simulink library "ddm"  (R2021b)
settings: Solver=VariableStepAuto  StartTime=0.0  StopTime=10.0  RelTol=1e-3
undefined symbols (not defined in the file or in its folder): ENUM_ADASACCSTA_ERROR, ENUM_ADASACCSTA_OFF, ENUM_ADASACCSTA_STANDBY, ENUM_ADASISASTA_OFF, ENUM_ALLOWMOV_ALLOWREADY, ENUM_APS, ENUM_BRKSTA_ERROR, ENUM_BRKSTA_OFF, ENUM_BRKSTA_ON, ENUM_CHGPREACTERRSTA_OBCPRE, ENUM_DCDCFAULTSTA_ANYFAULTLV1, ENUM_DCDCFAULTSTA_ANYFAULTLV2, ENUM_DRIVETRAIN_AWD, ENUM_DRIVETRAIN_FWD, ENUM_DRIVETRAIN_RWD, ENUM_DRSEATSTA_INVALID, ENUM_EDUDRTSTA_NORMAL, ENUM_EPBSTA_APPLIED, ENUM_EPBSTA_RELEASED, ENUM_HVBATTREADYPRE_READY, ENUM_MCUWARN_LV0, ENUM_MCUWARN_LV1, ENUM_MCUWARN_LV2, ENUM_MCUWARN_LV3, ENUM_MCUWARN_NOERROR, ENUM_OBCFAULTSTA_ANYFAULT, ENUM_PAS_R2F2, ENUM_PDFAULT_BATTPDFAIL, ENUM_PDFAULT_DCDCDISABLE, ENUM_PDFAULT_MCUDISABLE, ENUM_PDFAULT_MCUDISCHRG, ENUM_POWERSTA_OFF, ENUM_POWERSTA_ON, ENUM_POWERSTA_READY, ENUM_POWERSTA_STANDBY, ENUM_PRESSINDI_LOW, ENUM_PUFAULT_BATTUPFAIL, ENUM_PUFAULT_DCDCENABLEFAIL, ENUM_PUFAULT_PRECHRGCHKFAIL, ENUM_PUFAULT_SAFETYCHKFAIL, ENUM_PUSTATE_COMPLETED, ENUM_PWRSTASW_OFF, ENUM_PWRSTASW_OFFA, ENUM_PWRSTASW_OFFCHVCHRG, ENUM_PWRSTASW_OFFCLVCHRG, ENUM_PWRSTASW_ON, ENUM_PWRSTASW_ONHVCHRG, ENUM_PWRSTASW_READY, ENUM_PWRSTASW_STANDBY, ENUM_RANGESTA_12IN, ENUM_RANGESTA_12OUT, ENUM_SHIFTCOMMAND_D, ENUM_SHIFTCOMMAND_N, ENUM_SHIFTCOMMAND_P, ENUM_SHIFTCOMMAND_R, ENUM_ZONEMALFUNLV_1ST, ENUM_ZONEMALFUNLV_2ND, ENUM_ZONEMALFUNLV_3RD, ENUM_ZONEMALFUNLV_4TH, ENUM_ZONESPDCTRLMODE_ACC ... (+832)
libraries: hcu_lib x738, $bdroot x26, simulink x7
(part 5 of 25)

== system ddm/DDM/DDM/PMM/Brake switch signal abnormal ==
  task_time_s : Inport
  VPMM_PwrStaSW_enum : Inport  Port=2
  VPMM_PowerSta_enum : Inport  Port=3
  VINP_BrakeSWGPIO_flg : Inport  Port=4
  VINP_BrakeLampSW_flg : Inport  Port=5
  VDDM_ESC5NoComCFS_flg : Inport  Port=6
  VDDM_ESC5RCErrCFS_flg : Inport  Port=7
  VDDM_ESC5CSErrCFS_flg : Inport  Port=8
  VINP_DrStdAErrSta_enum : Inport  Port=9
  VINP_BrkSWSta_flg : Inport  Port=10
  VDDM_ESC7NoComCFS_flg : Inport  Port=11
  VDDM_ESC7RCErrCFS_flg : Inport  Port=12
  VDDM_ESC7CSErrCFS_flg : Inport  Port=13
  VINP_BrkPedalPosSta_enum : Inport  Port=14
  VINP_BrkPedalPos_pct : Inport  Port=15
  DTC_clear_request : Inport  Port=16
  Brake switch signal abnormal : Subsystem
  Brake switch signal abnormal and no backup signal : Subsystem
  Constant : Constant  Value=FALSE
  Constant1 : Constant  Value=ENUM_BRKSTA_ERROR
  Constant2 : Constant  Value=ENUM_BRKSTA_ON
  Constant3 : Constant  Value=ENUM_BRKSTA_OFF
  Constant4 : Constant  Value=FALSE
  Constant5 : Constant  Value=ENUM_BRKSTA_ERROR
  Constant6 : Constant  Value=ENUM_BRKSTA_ON
  Constant7 : Constant  Value=ENUM_BRKSTA_OFF
  Constant8 : Constant  Value=KDDM_BrkPedalPos_pct
  Equal : RelationalOperator  Operator===  OutDataTypeStr=boolean  RndMeth=Simplest
  Equal1 : RelationalOperator  Operator===  OutDataTypeStr=boolean  RndMeth=Simplest
  Equal2 : RelationalOperator  OutDataTypeStr=boolean  RndMeth=Simplest
  Logical Operator : Logic  Operator=OR  Inputs=4  AllPortsSameDT=off  OutDataTypeStr=boolean
  Logical Operator1 : Logic  Operator=OR  Inputs=4  AllPortsSameDT=off  OutDataTypeStr=boolean
  Subsystem : Subsystem
  Switch{,1..3} (4 alike) : Switch  Criteria=u2 > Threshold
  VDDM_BrkSWErrDTC_raw32 : Outport
  VDDM_BrkSWNoBacDTC_raw32 : Outport  Port=2
  VDDM_BrakeSW_enum : Outport  Port=3
  VDDM_CANBrkSW2Sta_enum : Outport  Port=4
  VDDM_BrkPedalPosSta_enum : Outport  Port=5
  VDDM_EDriveSysErrBrake_flg : Outport  Port=6
  VDDM_VCUBrkSWSta_flg : Outport  Port=7
  wires:
  [VPMM_PwrStaSW_enum] -> Brake switch signal abnormal and no backup signal/2(VPMM_PowerSta_enum)
  [VPMM_PowerSta_enum] -> Brake switch signal abnormal and no backup signal/3(VPMM_PwrStaSW_enum)
  [task_time_s] -> Brake switch signal abnormal and no backup signal/1(task_time_s)
  [VPMM_PowerSta_enum] -> Brake switch signal abnormal/3(VPMM_PwrStaSW_enum)
  [VPMM_PwrStaSW_enum] -> Brake switch signal abnormal/2(VPMM_PowerSta_enum)
  [task_time_s] -> Brake switch signal abnormal/1(task_time_s)
  VPMM_PowerSta_enum/1 -> [VPMM_PowerSta_enum]
  VPMM_PwrStaSW_enum/1 -> [VPMM_PwrStaSW_enum]
  task_time_s/1 -> [task_time_s]
  VINP_DrStdAErrSta_enum/1 -> Equal/1
  Constant/1 -> Equal/2
  VDDM_ESC5CSErrCFS_flg/1 -> Logical Operator/3
  VDDM_ESC5RCErrCFS_flg/1 -> Logical Operator/2
  VDDM_ESC5NoComCFS_flg/1 -> Logical Operator/1
  Equal/1 -> Logical Operator/4
  Switch1/1 -> Switch/3
  Logical Operator/1 -> Switch/2
  Constant1/1 -> Switch/1
  VINP_BrkSWSta_flg/1 -> Switch1/2
  Constant2/1 -> Switch1/1
  Constant3/1 -> Switch1/3
  Constant7/1 -> Switch3/3
  Constant6/1 -> Switch3/1
  Constant5/1 -> Switch2/1
  Logical Operator1/1 -> Switch2/2
  Switch3/1 -> Switch2/3
  Equal1/1 -> Logical Operator1/4
  VDDM_ESC7NoComCFS_flg/1 -> Logical Operator1/1
  VDDM_ESC7RCErrCFS_flg/1 -> Logical Operator1/2
  VDDM_ESC7CSErrCFS_flg/1 -> Logical Operator1/3
  Constant4/1 -> Equal1/2
  VINP_BrkPedalPosSta_enum/1 -> Equal1/1
  VINP_BrkPedalPos_pct/1 -> Equal2/1
  Constant8/1 -> Equal2/2
  Equal2/1 -> Switch3/2
  Brake switch signal abnormal/1(VDDM_BrkSWErrDTC_raw32) -> VDDM_BrkSWErrDTC_raw32/1
  Brake switch signal abnormal and no backup signal/1(VDDM_BrkSWNoBacDTC_raw32) -> VDDM_BrkSWNoBacDTC_raw32/1
  Switch/1 -> [VDDM_CANBrkSW2Sta_enum]
  Switch2/1 -> [VDDM_BrkPedalPosSta_enum]
  [VDDM_BrkPedalPosSta_enum] -> VDDM_BrkPedalPosSta_enum/1
  [VDDM_CANBrkSW2Sta_enum] -> VDDM_CANBrkSW2Sta_enum/1
  [VDDM_BrakeSW_enum] -> VDDM_BrakeSW_enum/1
  Brake switch signal abnormal/2(VDDM_EDriveSysErrBrake_flg) -> VDDM_EDriveSysErrBrake_flg/1
  Brake switch signal abnormal and no backup signal/2(VDDM_VCUBrkSWSta_flg) -> VDDM_VCUBrkSWSta_flg/1
  DTC_clear_request/1 -> [DTC_clear_request]
  [DTC_clear_request] -> Brake switch signal abnormal/6(DTC_clear_request)
  [DTC_clear_request] -> Brake switch signal abnormal and no backup signal/6(DTC_clear_request)
  [VDDM_CANBrkSW2Sta_enum] -> Subsystem/1(VDDM_CANBSW2S_enum)
  [VDDM_BrkPedalPosSta_enum] -> Subsystem/4(BrkPedalPos_enum)
  VINP_BrakeSWGPIO_flg/1 -> Subsystem/2(BrakeSW)
  VINP_BrakeLampSW_flg/1 -> Subsystem/3(Brake_Stop_Lamp)
  Subsystem/1(BrkSWErr) -> [BrkSWErr]
  Subsystem/4(VDDM_BrakeSW_enum) -> [VDDM_BrakeSW_enum]  "VDDM_BrakeSW_enum"
  Subsystem/2(BrkSWNoBac) -> [BrkSWNoBac]
  Subsystem/3(BrkSWPass) -> [BrkSWPass]
  [BrkSWErr] -> Brake switch signal abnormal/4(BrkSWErr)
  [BrkSWPass] -> Brake switch signal abnormal/5(BrkSWPass)
  [BrkSWNoBac] -> Brake switch signal abnormal and no backup signal/4(BrkSWNoBac)
  [BrkSWPass] -> Brake switch signal abnormal and no backup signal/5(BrkSWPass)

== system ddm/DDM/DDM/PMM/Comm err ==
  note: CAN1 ABM1
  note: CAN3 CCU2
  note: CAN3 CCU1
  note: CAN3 BMS1
  note: CAN3 BMS6
  note: CAN1 EPAS2
  task_time_s : Inport
  VPMM_PowerSta_enum : Inport  Port=2
  VPMM_PwrStaSW_enum : Inport  Port=3
  VDDM_C3BMS6RCChk_flg : Inport  Port=4
  VDDM_C3BMS6CSChk_flg : Inport  Port=5
  VDDM_C3BMS6LCChk_flg : Inport  Port=6
  VDDM_C3BMS1RCChk_flg : Inport  Port=7
  VDDM_C3BMS1CSChk_flg : Inport  Port=8
  VDDM_C3BMS1LCChk_flg : Inport  Port=9
  VDDM_C3CCU1RCChk_flg : Inport  Port=10
  VDDM_C3CCU1CSChk_flg : Inport  Port=11
  VDDM_C3CCU1LCChk_flg : Inport  Port=12
  VDDM_C3CCU2RCChk_flg : Inport  Port=13
  VDDM_C3CCU2CSChk_flg : Inport  Port=14
  VDDM_C3CCU2LCChk_flg : Inport  Port=15
  VDDM_C1ABM1RCChk_flg : Inport  Port=16
  VDDM_C1ABM1CSChk_flg : Inport  Port=17
  VDDM_C1ABM1LCChk_flg : Inport  Port=18
  No_CAN3_BUS_OFF : Inport  Port=19
  No_CAN1_BUS_OFF : Inport  Port=20
  DTC_clear_request : Inport  Port=21
  VDDM_C1EPAS2LCChk_flg : Inport  Port=22
  FDC lost communication with EPAS2 : Subsystem
  OR : Logic  Operator=OR  Inputs=3  AllPortsSameDT=off  OutDataTypeStr=boolean
  The CAN signal between VCU and ABM1 is discontinuous : Subsystem
  The CAN signal between VCU and ABM1 is incomplete : Subsystem
  The CAN signal between VCU and BMS1 is discontinuous : Subsystem
  The CAN signal between VCU and BMS1 is incomplete : Subsystem
  The CAN signal between VCU and BMS6 is discontinuous : Subsystem
  The CAN signal between VCU and BMS6 is incomplete : Subsystem
  The CAN signal between VCU and CCU1 is discontinuous : Subsystem
  The CAN signal between VCU and CCU1 is incomplete : Subsystem
  The CAN signal between VCU and CCU2 is discontinuous : Subsystem
  The CAN signal between VCU and CCU2 is incomplete : Subsystem
  VCU lost communication with ABM1 : Subsystem
  VCU lost communication with BMS1 : Subsystem
  VCU lost communication with BMS6 : Subsystem
  VCU lost communication with CCU1 : Subsystem
  VCU lost communication with CCU2 : Subsystem
  VDDM_C3BMS6RCDTC_raw32 : Outport
  VDDM_C3BMS6CSDTC_raw32 : Outport  Port=2
  VDDM_C3BMS6LCDTC_raw32 : Outport  Port=3
  VDDM_C3BMS1RCDTC_raw32 : Outport  Port=4
  VDDM_C3BMS1CSDTC_raw32 : Outport  Port=5
  VDDM_C3BMS1LCDTC_raw32 : Outport  Port=6
  VDDM_C3CCU1RCDTC_raw32 : Outport  Port=7
  VDDM_C3CCU1CSDTC_raw32 : Outport  Port=8
  VDDM_C3CCU1LCDTC_raw32 : Outport  Port=9
  VDDM_C3CCU2RCDTC_raw32 : Outport  Port=10
  VDDM_C3CCU2CSDTC_raw32 : Outport  Port=11
  VDDM_C3CCU2LCDTC_raw32 : Outport  Port=12
  VDDM_C1ABM1RCDTC_raw32 : Outport  Port=13
  VDDM_C1ABM1CSDTC_raw32 : Outport  Port=14
  VDDM_C1ABM1LCDTC_raw32 : Outport  Port=15
  VDDM_EDriveSysErrABMCAN_flg : Outport  Port=16
  VDDM_C3BMS6CSCFS_flg : Outport  Port=17
  VDDM_C3BMS6RCCFS_flg : Outport  Port=18
  VDDM_C3BMS6LCCFS_flg : Outport  Port=19
  VDDM_C3CCU2CSCFS_flg : Outport  Port=20
  VDDM_C3CCU2LCCFS_flg : Outport  Port=21
  VDDM_C3CCU2RCCFS_flg : Outport  Port=22
  VDDM_C1EPAS2LCDTC_raw32 : Outport  Port=23
  wires:
  [VDDM_C3CCU2LCCFS_flg] -> The CAN signal between VCU and CCU2 is incomplete/5(VDDM_C3CCU2LCCFS_flg)
  [VPMM_PwrStaSW_enum] -> The CAN signal between VCU and BMS6 is incomplete/3(VPMM_PwrStaSW_enum)
  [VPMM_PwrStaSW_enum] -> VCU lost communication with CCU2/3(VPMM_PwrStaSW_enum)
  [task_time_s] -> VCU lost communication with BMS6/1(task_time_s)
  [task_time_s] -> The CAN signal between VCU and CCU2 is discontinuous/1(task_time_s)
  [task_time_s] -> The CAN signal between VCU and BMS6 is discontinuous/1(task_time_s)
  [VPMM_PwrStaSW_enum] -> VCU lost communication with ABM1/3(VPMM_PwrStaSW_enum)
  VCU lost communication with CCU2/2(VDDM_C3CCU2LCCFS_flg) -> [VDDM_C3CCU2LCCFS_flg]
  [task_time_s] -> VCU lost communication with ABM1/1(task_time_s)
  [task_time_s] -> The CAN signal between VCU and BMS1 is incomplete/1(task_time_s)
  [VPMM_PwrStaSW_enum] -> VCU lost communication with BMS6/3(VPMM_PwrStaSW_enum)
  [VPMM_PowerSta_enum] -> VCU lost communication with ABM1/2(VPMM_PowerSta_enum)
  [VPMM_PwrStaSW_enum] -> The CAN signal between VCU and ABM1 is discontinuous/3(VPMM_PwrStaSW_enum)
  [VPMM_PowerSta_enum] -> The CAN signal between VCU and BMS6 is discontinuous/2(VPMM_PowerSta_enum)
  [task_time_s] -> VCU lost communication with CCU2/1(task_time_s)
  VCU lost communication with ABM1/2(VDDM_C1ABM1LCCFS_flg) -> [VDDM_C1ABM1LCCFS_flg]
  [VPMM_PwrStaSW_enum] -> The CAN signal between VCU and ABM1 is incomplete/3(VPMM_PwrStaSW_enum)
  VDDM_C1ABM1LCChk_flg/1 -> VCU lost communication with ABM1/4(VDDM_C1ABM1LCChk_flg)
  [task_time_s] -> The CAN signal between VCU and BMS6 is incomplete/1(task_time_s)
  [VDDM_C1ABM1LCCFS_flg] -> The CAN signal between VCU and ABM1 is discontinuous/5(VDDM_C1ABM1LCCFS_flg)
  [task_time_s] -> The CAN signal between VCU and CCU1 is incomplete/1(task_time_s)
  VCU lost communication with BMS1/2(VDDM_C3BMS1LCCFS_flg) -> [VDDM_C3BMS1LCCFS_flg]
  [VPMM_PowerSta_enum] -> The CAN signal between VCU and CCU2 is discontinuous/2(VPMM_PowerSta_enum)
  [VPMM_PowerSta_enum] -> VCU lost communication with BMS1/2(VPMM_PowerSta_enum)
  [task_time_s] -> The CAN signal between VCU and BMS1 is discontinuous/1(task_time_s)
  [VPMM_PwrStaSW_enum] -> The CAN signal between VCU and BMS1 is discontinuous/3(VPMM_PwrStaSW_enum)
  [VDDM_C3CCU1LCCFS_flg] -> The CAN signal between VCU and CCU1 is discontinuous/5(VDDM_C3CCU1LCCFS_flg)
  [VPMM_PowerSta_enum] -> The CAN signal between VCU and BMS6 is incomplete/2(VPMM_PowerSta_enum)
  [VDDM_C3CCU2LCCFS_flg] -> The CAN signal between VCU and CCU2 is discontinuous/5(VDDM_C3CCU2LCCFS_flg)
  [VPMM_PwrStaSW_enum] -> VCU lost communication with BMS1/3(VPMM_PwrStaSW_enum)
  [No_CAN3_BUS_OFF] -> The CAN signal between VCU and BMS6 is incomplete/6(No_CAN3_BUS_OFF)
  [VPMM_PowerSta_enum] -> The CAN signal between VCU and BMS1 is discontinuous/2(VPMM_PowerSta_enum)
  [task_time_s] -> The CAN signal between VCU and ABM1 is incomplete/1(task_time_s)
  VDDM_C3BMS1LCChk_flg/1 -> VCU lost communication with BMS1/4(VDDM_C3BMS1LCChk_flg)
  [VPMM_PowerSta_enum] -> The CAN signal between VCU and BMS1 is incomplete/2(VPMM_PowerSta_enum)
  [VDDM_C3BMS1LCCFS_flg] -> The CAN signal between VCU and BMS1 is incomplete/5(VDDM_C3BMS1LCCFS_flg)
  [task_time_s] -> VCU lost communication with CCU1/1(task_time_s)
  [VPMM_PowerSta_enum] -> The CAN signal between VCU and CCU2 is incomplete/2(VPMM_PowerSta_enum)
  [VPMM_PwrStaSW_enum] -> The CAN signal between VCU and BMS1 is incomplete/3(VPMM_PwrStaSW_enum)
  [VPMM_PowerSta_enum] -> VCU lost communication with BMS6/2(VPMM_PowerSta_enum)
  [task_time_s] -> VCU lost communication with BMS1/1(task_time_s)
  [No_CAN3_BUS_OFF] -> The CAN signal between VCU and BMS1 is discontinuous/6(No_CAN3_BUS_OFF)
  VCU lost communication with CCU1/2(VDDM_C3CCU1LCCFS_flg) -> [VDDM_C3CCU1LCCFS_flg]
  [No_CAN3_BUS_OFF] -> The CAN signal between VCU and BMS6 is discontinuous/6(No_CAN3_BUS_OFF)
  [VPMM_PowerSta_enum] -> The CAN signal between VCU and CCU1 is incomplete/2(VPMM_PowerSta_enum)
  [task_time_s] -> The CAN signal between VCU and CCU1 is discontinuous/1(task_time_s)
  [VPMM_PwrStaSW_enum] -> The CAN signal between VCU and BMS6 is discontinuous/3(VPMM_PwrStaSW_enum)
  [VPMM_PwrStaSW_enum] -> The CAN signal between VCU and CCU1 is discontinuous/3(VPMM_PwrStaSW_enum)
  [VPMM_PwrStaSW_enum] -> The CAN signal between VCU and CCU1 is incomplete/3(VPMM_PwrStaSW_enum)
  [VPMM_PowerSta_enum] -> VCU lost communication with CCU1/2(VPMM_PowerSta_enum)
  [VPMM_PwrStaSW_enum] -> VCU lost communication with CCU1/3(VPMM_PwrStaSW_enum)
  [VDDM_C3CCU1LCCFS_flg] -> The CAN signal between VCU and CCU1 is incomplete/5(VDDM_C3CCU1LCCFS_flg)
  [VPMM_PowerSta_enum] -> The CAN signal between VCU and CCU1 is discontinuous/2(VPMM_PowerSta_enum)
  VCU lost communication with BMS6/2(VDDM_C3BMS6LCCFS_flg) -> [VDDM_C3BMS6LCCFS_flg]
  [VPMM_PwrStaSW_enum] -> The CAN signal between VCU and CCU2 is discontinuous/3(VPMM_PwrStaSW_enum)
  [task_time_s] -> The CAN signal between VCU and CCU2 is incomplete/1(task_time_s)
  [VPMM_PowerSta_enum] -> VCU lost communication with CCU2/2(VPMM_PowerSta_enum)
  [VPMM_PowerSta_enum] -> The CAN signal between VCU and ABM1 is incomplete/2(VPMM_PowerSta_enum)
  [VPMM_PwrStaSW_enum] -> The CAN signal between VCU and CCU2 is incomplete/3(VPMM_PwrStaSW_enum)
  [VDDM_C1ABM1LCCFS_flg] -> The CAN signal between VCU and ABM1 is incomplete/5(VDDM_C1ABM1LCCFS_flg)
  [task_time_s] -> The CAN signal between VCU and ABM1 is discontinuous/1(task_time_s)
  [VPMM_PowerSta_enum] -> The CAN signal between VCU and ABM1 is discontinuous/2(VPMM_PowerSta_enum)
  VDDM_C3CCU2CSChk_flg/1 -> The CAN signal between VCU and CCU2 is incomplete/4(VDDM_C3CCU2CSChk_flg)
  VDDM_C3BMS1RCChk_flg/1 -> The CAN signal between VCU and BMS1 is discontinuous/4(VDDM_C3BMS1RCChk_flg)
  VDDM_C3CCU1LCChk_flg/1 -> VCU lost communication with CCU1/4(VDDM_C3CCU1LCChk_flg)
  VDDM_C3CCU1RCChk_flg/1 -> The CAN signal between VCU and CCU1 is discontinuous/4(VDDM_C3CCU1RCChk_flg)
  VDDM_C1ABM1RCChk_flg/1 -> The CAN signal between VCU and ABM1 is discontinuous/4(VDDM_C1ABM1RCChk_flg)
  VDDM_C1ABM1CSChk_flg/1 -> The CAN signal between VCU and ABM1 is incomplete/4(VDDM_C1ABM1CSChk_flg)
  VDDM_C3BMS1CSChk_flg/1 -> The CAN signal between VCU and BMS1 is incomplete/4(VDDM_C3BMS1CSChk_flg)
  VDDM_C3CCU1CSChk_flg/1 -> The CAN signal between VCU and CCU1 is incomplete/4(VDDM_C3CCU1CSChk_flg)
  VDDM_C3CCU2LCChk_flg/1 -> VCU lost communication with CCU2/4(VDDM_C3CCU2LCChk_flg)
  VDDM_C3CCU2RCChk_flg/1 -> The CAN signal between VCU and CCU2 is discontinuous/4(VDDM_C3CCU2RCChk_flg)
  VPMM_PowerSta_enum/1 -> [VPMM_PowerSta_enum]
  VPMM_PwrStaSW_enum/1 -> [VPMM_PwrStaSW_enum]
  task_time_s/1 -> [task_time_s]
  VDDM_C3BMS6RCChk_flg/1 -> The CAN signal between VCU and BMS6 is discontinuous/4(VDDM_C3BMS6RCChk_flg)
  VDDM_C3BMS6CSChk_flg/1 -> The CAN signal between VCU and BMS6 is incomplete/4(VDDM_C3BMS6CSChk_flg)
  VDDM_C3BMS6LCChk_flg/1 -> VCU lost communication with BMS6/4(VDDM_C3BMS6LCChk_flg)
  [DTC_clear_request] -> The CAN signal between VCU and BMS6 is discontinuous/7(DTC_clear_request)
  [DTC_clear_request] -> The CAN signal between VCU and BMS6 is incomplete/7(DTC_clear_request)
  [VDDM_C3BMS6LCCFS_flg] -> The CAN signal between VCU and BMS6 is discontinuous/5(VDDM_C3BMS6LCCFS_flg)
  [VDDM_C3BMS6LCCFS_flg] -> The CAN signal between VCU and BMS6 is incomplete/5(VDDM_C3BMS6LCCFS_flg)
  [No_CAN3_BUS_OFF] -> VCU lost communication with BMS6/5(No_CAN3_BUS_OFF)
  [DTC_clear_request] -> VCU lost communication with BMS6/6(DTC_clear_request)
  [DTC_clear_request] -> The CAN signal between VCU and BMS1 is discontinuous/7(DTC_clear_request)
  [VDDM_C3BMS1LCCFS_flg] -> The CAN signal between VCU and BMS1 is discontinuous/5(VDDM_C3BMS1LCCFS_flg)
  [No_CAN3_BUS_OFF] -> The CAN signal between VCU and BMS1 is incomplete/6(No_CAN3_BUS_OFF)
  [DTC_clear_request] -> The CAN signal between VCU and BMS1 is incomplete/7(DTC_clear_request)
  [No_CAN3_BUS_OFF] -> VCU lost communication with BMS1/5(No_CAN3_BUS_OFF)
  [DTC_clear_request] -> VCU lost communication with BMS1/6(DTC_clear_request)
  [No_CAN3_BUS_OFF] -> The CAN signal between VCU and CCU1 is discontinuous/6(No_CAN3_BUS_OFF)
  [DTC_clear_request] -> The CAN signal between VCU and CCU1 is discontinuous/7(DTC_clear_request)
  [No_CAN3_BUS_OFF] -> The CAN signal between VCU and CCU1 is incomplete/6(No_CAN3_BUS_OFF)
  [DTC_clear_request] -> The CAN signal between VCU and CCU1 is incomplete/7(DTC_clear_request)
  [No_CAN3_BUS_OFF] -> VCU lost communication with CCU1/5(No_CAN3_BUS_OFF)
  [DTC_clear_request] -> VCU lost communication with CCU1/6(DTC_clear_request)
  [No_CAN3_BUS_OFF] -> The CAN signal between VCU and CCU2 is discontinuous/6(No_CAN3_BUS_OFF)
  [DTC_clear_request] -> The CAN signal between VCU and CCU2 is discontinuous/7(DTC_clear_request)
  [No_CAN3_BUS_OFF] -> The CAN signal between VCU and CCU2 is incomplete/6(No_CAN3_BUS_OFF)
  [DTC_clear_request] -> The CAN signal between VCU and CCU2 is incomplete/7(DTC_clear_request)
  [No_CAN3_BUS_OFF] -> VCU lost communication with CCU2/5(No_CAN3_BUS_OFF)
  [DTC_clear_request] -> VCU lost communication with CCU2/6(DTC_clear_request)
  [No_CAN1_BUS_OFF] -> The CAN signal between VCU and ABM1 is discontinuous/6(No_CAN1_BUS_OFF)
  [DTC_clear_request] -> The CAN signal between VCU and ABM1 is discontinuous/7(DTC_clear_request)
  [No_CAN1_BUS_OFF] -> The CAN signal between VCU and ABM1 is incomplete/6(No_CAN1_BUS_OFF)
  [DTC_clear_request] -> The CAN signal between VCU and ABM1 is incomplete/7(DTC_clear_request)
  The CAN signal between VCU and ABM1 is discontinuous/2(RC_EDriveSysErr_VCUErr_flg) -> [VDDM_EDriveSysErrABMRC_flg]
  The CAN signal between VCU and ABM1 is incomplete/2(CS_EDriveSysErr_VCUErr_flg) -> [VDDM_EDriveSysErrABMCS_flg]
  [No_CAN1_BUS_OFF] -> VCU lost communication with ABM1/5(No_CAN1_BUS_OFF)
  [DTC_clear_request] -> VCU lost communication with ABM1/6(DTC_clear_request)
  VCU lost communication with ABM1/3(LC_EDriveSysErr_VCUErr_flg) -> [VDDM_EDriveSysErrABMLC_flg]
  [VDDM_EDriveSysErrABMCS_flg] -> OR/2
  [VDDM_EDriveSysErrABMRC_flg] -> OR/1
  [VDDM_EDriveSysErrABMLC_flg] -> OR/3
  OR/1 -> VDDM_EDriveSysErrABMCAN_flg/1
  No_CAN3_BUS_OFF/1 -> [No_CAN3_BUS_OFF]
  No_CAN1_BUS_OFF/1 -> [No_CAN1_BUS_OFF]
  DTC_clear_request/1 -> [DTC_clear_request]
  The CAN signal between VCU and BMS6 is discontinuous/1(VDDM_C3BMS6RCDTC_raw32) -> VDDM_C3BMS6RCDTC_raw32/1
  The CAN signal between VCU and BMS6 is incomplete/1(VDDM_C3BMS6CSDTC_raw32) -> VDDM_C3BMS6CSDTC_raw32/1
  The CAN signal between VCU and BMS1 is discontinuous/1(VDDM_C3BMS1RCDTC_raw32) -> VDDM_C3BMS1RCDTC_raw32/1
  The CAN signal between VCU and BMS1 is incomplete/1(VDDM_C3BMS1CSDTC_raw32) -> VDDM_C3BMS1CSDTC_raw32/1
  VCU lost communication with BMS1/1(VDDM_C3BMS1LCDTC_raw32) -> VDDM_C3BMS1LCDTC_raw32/1
  The CAN signal between VCU and CCU1 is incomplete/1(VDDM_C3CCU1CSDTC_raw32) -> VDDM_C3CCU1CSDTC_raw32/1
  VCU lost communication with CCU1/1(VDDM_C3CCU1LCDTC_raw32) -> VDDM_C3CCU1LCDTC_raw32/1
  The CAN signal between VCU and CCU2 is discontinuous/1(VDDM_C3CCU2RCDTC_raw32) -> VDDM_C3CCU2RCDTC_raw32/1
  The CAN signal between VCU and CCU2 is incomplete/1(VDDM_C3CCU2CSDTC_raw32) -> VDDM_C3CCU2CSDTC_raw32/1
  VCU lost communication with CCU2/1(VDDM_C3CCU2LCDTC_raw32) -> VDDM_C3CCU2LCDTC_raw32/1
  The CAN signal between VCU and ABM1 is discontinuous/1(VDDM_C1ABM1RCDTC_raw32) -> VDDM_C1ABM1RCDTC_raw32/1
  The CAN signal between VCU and ABM1 is incomplete/1(VDDM_C1ABM1CSDTC_raw32) -> VDDM_C1ABM1CSDTC_raw32/1
  VCU lost communication with ABM1/1(VDDM_C1ABM1LCDTC_raw32) -> VDDM_C1ABM1LCDTC_raw32/1
  VCU lost communication with BMS6/1(VDDM_C3BMS6LCDTC_raw32) -> VDDM_C3BMS6LCDTC_raw32/1
  The CAN signal between VCU and CCU1 is discontinuous/1(VDDM_C3CCU1RCDTC_raw32) -> VDDM_C3CCU1RCDTC_raw32/1
  The CAN signal between VCU and BMS6 is incomplete/2(VDDM_C3BMS6CSCFS_flg) -> VDDM_C3BMS6CSCFS_flg/1
  [VDDM_C3BMS6LCCFS_flg] -> VDDM_C3BMS6LCCFS_flg/1
  The CAN signal between VCU and BMS6 is discontinuous/2(VDDM_C3BMS6RCCFS_flg) -> VDDM_C3BMS6RCCFS_flg/1
  The CAN signal between VCU and CCU2 is incomplete/2(VDDM_C3CCU2CSCFS_flg) -> VDDM_C3CCU2CSCFS_flg/1
  [VDDM_C3CCU2LCCFS_flg] -> VDDM_C3CCU2LCCFS_flg/1
  The CAN signal between VCU and CCU2 is discontinuous/2(VDDM_C3CCU2RCCFS_flg) -> VDDM_C3CCU2RCCFS_flg/1
  FDC lost communication with EPAS2/1(VDDM_C1EPAS2LCDTC_raw32) -> VDDM_C1EPAS2LCDTC_raw32/1
  [DTC_clear_request] -> FDC lost communication with EPAS2/6(DTC_clear_request)
  [No_CAN1_BUS_OFF] -> FDC lost communication with EPAS2/5(No_CAN1_BUS_OFF)
  VDDM_C1EPAS2LCChk_flg/1 -> FDC lost communication with EPAS2/4(VDDM_C1EPAS2LCChk_flg)
  [VPMM_PwrStaSW_enum] -> FDC lost communication with EPAS2/3(VPMM_PwrStaSW_enum)
  [VPMM_PowerSta_enum] -> FDC lost communication with EPAS2/2(VPMM_PowerSta_enum)
  FDC lost communication with EPAS2/2(VDDM_C1EPAS2LCCFS_flg) -> [VDDM_C1EPAS2LCCFS_flg]
  [task_time_s] -> FDC lost communication with EPAS2/1(task_time_s)

== system ddm/DDM/DDM/PMM/Fault level ==
  task_time_s : Inport
  VPMM_PwrStaSW_enum : Inport  Port=2
  VPMM_PowerSta_enum : Inport  Port=3
  VINP_BMSWarn1_flg : Inport  Port=4
  VINP_BMSWarn2_flg : Inport  Port=5
  VINP_BMSWarn3_flg : Inport  Port=6
  VINP_BMSWarn4_flg : Inport  Port=7
  VINP_BMSWarn5_flg : Inport  Port=8
  VINP_BMSWarn6_flg : Inport  Port=9
  VINP_BMSWarn7_flg : Inport  Port=10
  VINP_BMSWarn8_flg : Inport  Port=11
  VINP_DCDCFaultSta_enum : Inport  Port=12
  VPMM_DrivetrainSelect_enum : Inport  Port=13
  VDDM_C3BMS6LCCFS_flg : Inport  Port=14
  VDDM_C3CCU2LCCFS_flg : Inport  Port=15
  VDDM_MCUF1NoComCFS_flg : Inport  Port=16
  VDDM_MCUR1NoComCFS_flg : Inport  Port=17
  VINP_MCUWarnF_enum : Inport  Port=18
  VINP_MCUWarnR_enum : Inport  Port=19
  VINP_OBCFaultSta_enum : Inport  Port=20
  DTC_clear_request : Inport  Port=21
  No_CAN3_BUS_OFF : Inport  Port=22
  Fault level 1 subsystem error : Subsystem
  Fault level 2 subsystem error : Subsystem
  Fault level 3 subsystem error : Subsystem
  Fault level 4 subsystem error : Subsystem
  VDDM_Lv1ErrDTC_raw32 : Outport
  VDDM_Lv2ErrCFS_flg : Outport  Port=2
  VDDM_Lv3ErrDTC_raw32 : Outport  Port=3
  VDDM_Lv4ErrDTC_raw32 : Outport  Port=4
  wires:
  task_time_s/1 -> [task_time_s]
  VPMM_PwrStaSW_enum/1 -> [VPMM_PwrStaSW_enum]
  VPMM_PowerSta_enum/1 -> [VPMM_PowerSta_enum]
  [task_time_s] -> Fault level 1 subsystem error/1(task_time_s)
  [VPMM_PwrStaSW_enum] -> Fault level 1 subsystem error/2(VPMM_PowerSta_enum)
  [VPMM_PowerSta_enum] -> Fault level 1 subsystem error/3(VPMM_PwrStaSW_enum)
  [VPMM_PowerSta_enum] -> Fault level 2 subsystem error/3(VPMM_PwrStaSW_enum)
  [VPMM_PwrStaSW_enum] -> Fault level 2 subsystem error/2(VPMM_PowerSta_enum)
  [task_time_s] -> Fault level 2 subsystem error/1(task_time_s)
  VINP_DCDCFaultSta_enum/1 -> [VINP_DCDCFaultSta_enum]
  [VINP_DCDCFaultSta_enum] -> Fault level 2 subsystem error/10(VINP_DCDCFaultSta_enum)
  [VINP_DCDCFaultSta_enum] -> Fault level 1 subsystem error/11(VINP_DCDCFaultSta_enum)
  [task_time_s] -> Fault level 3 subsystem error/1(task_time_s)
  [VPMM_PwrStaSW_enum] -> Fault level 3 subsystem error/2(VPMM_PowerSta_enum)
  [VPMM_PowerSta_enum] -> Fault level 3 subsystem error/3(VPMM_PwrStaSW_enum)
  VPMM_DrivetrainSelect_enum/1 -> [VPMM_DrivetrainSelect_enum]
  [VPMM_DrivetrainSelect_enum] -> Fault level 1 subsystem error/15(VPMM_DrivetrainSelect_enum)
  [task_time_s] -> Fault level 4 subsystem error/1(task_time_s)
  [VPMM_PwrStaSW_enum] -> Fault level 4 subsystem error/2(VPMM_PowerSta_enum)
  [VPMM_PowerSta_enum] -> Fault level 4 subsystem error/3(VPMM_PwrStaSW_enum)
  VDDM_C3BMS6LCCFS_flg/1 -> [VDDM_C3BMS6LCCFS_flg]
  [VDDM_C3BMS6LCCFS_flg] -> Fault level 1 subsystem error/4(VDDM_C3BMS6LCCFS_flg)
  [VDDM_C3BMS6LCCFS_flg] -> Fault level 2 subsystem error/4(VDDM_C3BMS6LCCFS_flg)
  VDDM_MCUR1NoComCFS_flg/1 -> [VDDM_MCUR1NoComCFS_flg]
  VDDM_MCUF1NoComCFS_flg/1 -> [VDDM_MCUF1NoComCFS_flg]
  [VDDM_MCUR1NoComCFS_flg] -> Fault level 1 subsystem error/7(VDDM_MCUR1NoComCFS_flg)
  [VDDM_MCUF1NoComCFS_flg] -> Fault level 1 subsystem error/6(VDDM_MCUF1NoComCFS_flg)
  VINP_BMSWarn5_flg/1 -> Fault level 2 subsystem error/9(VINP_BMSWarn5_flg)
  VINP_BMSWarn4_flg/1 -> Fault level 2 subsystem error/8(VINP_BMSWarn4_flg)
  [VDDM_MCUR1NoComCFS_flg] -> Fault level 2 subsystem error/7(VDDM_MCUR1NoComCFS_flg)
  [VDDM_MCUF1NoComCFS_flg] -> Fault level 2 subsystem error/6(VDDM_MCUF1NoComCFS_flg)
  [VDDM_MCUF1NoComCFS_flg] -> Fault level 3 subsystem error/5(VDDM_MCUF1NoComCFS_flg)
  [VDDM_MCUR1NoComCFS_flg] -> Fault level 3 subsystem error/6(VDDM_MCUR1NoComCFS_flg)
  [VDDM_C3BMS6LCCFS_flg] -> Fault level 3 subsystem error/4(VDDM_C3BMS6LCCFS_flg)
  [VDDM_C3BMS6LCCFS_flg] -> Fault level 4 subsystem error/4(VDDM_C3BMS6LCCFS_flg)
  VINP_BMSWarn7_flg/1 -> Fault level 4 subsystem error/5(VINP_BMSWarn7_flg)
  VINP_BMSWarn8_flg/1 -> Fault level 4 subsystem error/6(VINP_BMSWarn8_flg)
  VINP_BMSWarn6_flg/1 -> Fault level 3 subsystem error/7(VINP_BMSWarn6_flg)
  VDDM_C3CCU2LCCFS_flg/1 -> [VDDM_C3CCU2LCCFS_flg]
  [VDDM_C3CCU2LCCFS_flg] -> Fault level 1 subsystem error/5(VDDM_C3CCU2LCCFS_flg)
  [VDDM_C3CCU2LCCFS_flg] -> Fault level 2 subsystem error/5(VDDM_C3CCU2LCCFS_flg)
  VINP_BMSWarn1_flg/1 -> Fault level 1 subsystem error/8(VINP_BMSWarn1_flg)
  VINP_BMSWarn2_flg/1 -> Fault level 1 subsystem error/9(VINP_BMSWarn2_flg)
  VINP_BMSWarn3_flg/1 -> Fault level 1 subsystem error/10(VINP_BMSWarn3_flg)
  VINP_MCUWarnF_enum/1 -> [VINP_MCUWarnF_enum]
  VINP_MCUWarnR_enum/1 -> [VINP_MCUWarnR_enum]
  VINP_OBCFaultSta_enum/1 -> [VINP_OBCFaultSta_enum]
  [VINP_OBCFaultSta_enum] -> Fault level 1 subsystem error/14(VINP_OBCFaultSta_enum)
  [VPMM_DrivetrainSelect_enum] -> Fault level 2 subsystem error/13(VPMM_DrivetrainSelect_enum)
  [VINP_MCUWarnF_enum] -> Fault level 2 subsystem error/11(VINP_MCUWarnF_enum)
  [VINP_MCUWarnR_enum] -> Fault level 2 subsystem error/12(VINP_MCUWarnR_enum)
  [VPMM_DrivetrainSelect_enum] -> Fault level 3 subsystem error/10(VPMM_DrivetrainSelect_enum)
  [VINP_MCUWarnR_enum] -> Fault level 3 subsystem error/9(VINP_MCUWarnR_enum)
  [VINP_MCUWarnF_enum] -> Fault level 3 subsystem error/8(VINP_MCUWarnF_enum)
  Fault level 1 subsystem error/1(VDDM_Lv1ErrDTC_raw32) -> VDDM_Lv1ErrDTC_raw32/1
  Fault level 2 subsystem error/1(VDDM_Lv2ErrDTC_raw32) -> VDDM_Lv2ErrCFS_flg/1
  Fault level 3 subsystem error/1(VDDM_Lv3ErrDTC_raw32) -> VDDM_Lv3ErrDTC_raw32/1
  Fault level 4 subsystem error/1(VDDM_Lv4ErrDTC_raw32) -> VDDM_Lv4ErrDTC_raw32/1
  [VINP_MCUWarnF_enum] -> Fault level 1 subsystem error/12(VINP_MCUWarnF_enum)
  [VINP_MCUWarnR_enum] -> Fault level 1 subsystem error/13(VINP_MCUWarnR_enum)
  No_CAN3_BUS_OFF/1 -> [No_CAN3_BUS_OFF]
  DTC_clear_request/1 -> [DTC_clear_request]
  [No_CAN3_BUS_OFF] -> Fault level 1 subsystem error/17(No_CAN3_BUS_OFF)
  [DTC_clear_request] -> Fault level 1 subsystem error/16(DTC_clear_request)
  [DTC_clear_request] -> Fault level 2 subsystem error/14(DTC_clear_request)
  [No_CAN3_BUS_OFF] -> Fault level 2 subsystem error/15(No_CAN3_BUS_OFF)
  [No_CAN3_BUS_OFF] -> Fault level 3 subsystem error/12(No_CAN3_BUS_OFF)
  [DTC_clear_request] -> Fault level 3 subsystem error/11(DTC_clear_request)
  [DTC_clear_request] -> Fault level 4 subsystem error/7(DTC_clear_request)
  [No_CAN3_BUS_OFF] -> Fault level 4 subsystem error/8(No_CAN3_BUS_OFF)

== system ddm/DDM/DDM/PMM/Key authentication failed ==
  note: Fail Safe Operation During Failure Detection
  note: Test Pass Criteria
  note: Diagnostics and Fault Handling
  note: Release Condition After Failure Decision
  note: Test Detection Criteria
  note: Fail Safe Operation After Failure Decision
  note: Release Condition During Failure Detection
  task_time_s : Inport
  VPMM_PowerSta_enum : Inport  Port=2
  VPMM_PwrStaSW_enum : Inport  Port=3
  VDDM_BrakeSW_enum : Inport  Port=4
  DTC_clear_request : Inport  Port=5
  VDKC_DKCAuthSta_enum : Inport  Port=6
  Constant11 : Constant  Value=KDDM_KeyAuthPassSW_flg
  Constant15 : Constant  Value=KDDM_KeyAuthCFSSW_flg
  Constant16 : Constant  Value=TRUE
  Constant19 : Constant  Value=ENUM_POWERSTA_OFF
  Constant{2,21,25,27} (4 alike) : Constant  Value=FALSE
  Constant20 : Constant  Value=KDDM_KeyAuthDFSSW_flg
  Constant23 : Constant  Value=TRUE
  Constant24 : Constant  Value=TRUE
  Constant26 : Constant  Value=ENUM_PWRSTASW_READY
  Constant3 : Constant  Value=ENUM_BRKSTA_ON
  Constant38 : Constant  Value=KDDM_KeyAuthDetTO_s
  Constant4 : Constant  Value=ENUM_PWRSTASW_READY
  Constant40 : Constant  Value=KDDM_KeyAuthDTC_cnt
  Constant43 : Constant  Value=KDDM_KeyAuthPassTO_s
  Constant44 : Constant  Value=KDDM_KeyAuthDetSW_flg
  Constant5 : Constant  Value=ENUM_BRKSTA_ON
  Constant7 : Constant  Value=KDDM_KeyAuthPassTO_s
  Constant8 : Constant  Value=KDDM_KeyAuthDTC_cnt
  DTC_Couter : hcu_lib/Basic_Blocks/DTC_Couter
  DTC_Info : hcu_lib/Basic_Blocks/DTC_Info
  Data Type Conversion1 : DataTypeConversion  OutDataTypeStr=uint8
  Equal{,2..3,5..6} (5 alike) : RelationalOperator  Operator===  OutDataTypeStr=boolean  RndMeth=Simplest
  Equal4 : RelationalOperator  OutDataTypeStr=boolean  RndMeth=Simplest
  Logical Operator{1..2,12,15,18..19} (6 alike) : Logic  AllPortsSameDT=off  OutDataTypeStr=boolean
  Logical Operator3 : Logic  Operator=OR  AllPortsSameDT=off  OutDataTypeStr=boolean
  Logical Operator6 : Logic  Operator=NOT  AllPortsSameDT=off  OutDataTypeStr=boolean
  Logical Operator8 : Logic  Operator=OR  AllPortsSameDT=off  OutDataTypeStr=boolean
  Relay : Relay  OnSwitchValue=ONE_INT  OffSwitchValue=ZERO_INT
  SR_Latch1 : Subsystem  mask(SR_Latch){}
      mask help: SR latch function.
  SR_Latch3 : hcu_lib/Basic_Blocks/SR_Latch
  SR_Latch4 : hcu_lib/Basic_Blocks/SR_Latch
  Switch{,2,4..6} (5 alike) : Switch  Criteria=u2 ~= 0
  Test Detection Criteria : hcu_lib/Basic_Blocks/Test Detection Criteria
  Timer1 : hcu_lib/Basic_Blocks/Timer
  VDDM_KeyAuthDTC_raw32 : Outport
  VDDM_EDriveSysErrKeyAuth_flg : Outport  Port=2
  wires:
  VPMM_PowerSta_enum/1 -> [VPMM_PowerSta_enum]
  VPMM_PwrStaSW_enum/1 -> [VPMM_PwrStaSW_enum]
  task_time_s/1 -> [task_time_s]
  VDDM_BrakeSW_enum/1 -> [VDDM_BrakeSW_enum]
  VDKC_DKCAuthSta_enum/1 -> [VDKC_DKCAuthSta_enum]
  Timer1/1 -> Equal4/1
  [VPMM_PwrStaSW_enum] -> Equal/1
  [task_time_s] -> Test Detection Criteria/2
  [VDDM_KeyAuthDTC_cnt] -> Relay/1
  Logical Operator3/1 -> Logical Operator15/1
  Constant40/1 -> Test Detection Criteria/3
  Constant43/1 -> Timer1/4
  Constant26/1 -> Equal/2
  Constant15/1 -> Logical Operator18/2
  Constant11/1 -> Logical Operator15/2
  Data Type Conversion1/1 -> [VDDM_KeyAuthDTC_cnt]  "VDDM_KeyAuthDTC_cnt"
  Logical Operator15/1 -> DTC_Couter/2
  Logical Operator6/1 -> Timer1/1
  Logical Operator12/1 -> [VDDM_KeyAuthDFS_flg]
  SR_Latch1/1(latched) -> [VDDM_KeyAuthPass_flg]
  [VDDM_KeyAuthCFS_flg] -> Switch/2
  Constant27/1 -> Switch5/3
  Constant24/1 -> Switch4/1
  Logical Operator19/1 -> DTC_Couter/1
  Equal/1 -> Logical Operator2/1
  Switch2/1 -> Timer1/2, Logical Operator6/1
  Logical Operator18/1 -> [VDDM_KeyAuthCFS_flg]
  [VDDM_KeyAuthCFSRls_flg] -> Logical Operator3/2
  Switch/1 -> [VDDM_EDriveSysErrKeyAuth_flg]
  DTC_Couter/2 -> Data Type Conversion1/1
  [VDDM_KeyAuthPass_flg] -> Logical Operator3/1
  [VPMM_PowerSta_enum] -> Equal5/1
  Constant16/1 -> Switch/1
  Logical Operator2/1 -> Switch5/2
  DTC_Couter/1 -> SR_Latch4/1
  Constant19/1 -> Equal5/2
  Logical Operator8/1 -> Switch4/2
  Switch4/1 -> [VDDM_KeyAuthCFSRls_flg]
  [VDDM_KeyAuthDet_flg] -> Logical Operator19/1
  Relay/1 -> SR_Latch3/1
  Constant21/1 -> Switch/3
  Constant20/1 -> Logical Operator12/1
  Test Detection Criteria/1 -> [VDDM_KeyAuthDet_flg]  "VDDM_KeyAuthDet_flg"
  SR_Latch4/1 -> Logical Operator18/1
  Constant8/1 -> DTC_Couter/3
  Constant25/1 -> Switch4/3
  Equal4/1 -> SR_Latch1/1(set)
  Constant44/1 -> Logical Operator19/2
  Constant7/1 -> Equal4/2
  Constant23/1 -> Switch2/3
  SR_Latch3/1 -> Logical Operator12/2
  Equal5/1 -> Logical Operator8/1
  [VDDM_KeyAuthCFSRls_flg] -> SR_Latch4/2
  [DTC_clear_request] -> Logical Operator8/2
  Equal2/1 -> Logical Operator2/2
  [VDDM_BrakeSW_enum] -> Equal2/1
  Constant3/1 -> Equal2/2
  [VDKC_DKCAuthSta_enum] -> Switch5/1
  [VPMM_PwrStaSW_enum] -> Equal3/1
  Equal3/1 -> Logical Operator1/1
  Logical Operator1/1 -> Switch2/2
  [VDDM_BrakeSW_enum] -> Equal6/1
  Constant5/1 -> Equal6/2
  [VDKC_DKCAuthSta_enum] -> Switch2/1
  Equal6/1 -> Logical Operator1/2
  Constant4/1 -> Equal3/2
  DTC_clear_request/1 -> [DTC_clear_request]
  [VDDM_EDriveSysErrKeyAuth_flg] -> VDDM_EDriveSysErrKeyAuth_flg/1
  [task_time_s] -> Timer1/3
  [VDDM_KeyAuthPass_flg] -> DTC_Info/2
  [VDDM_KeyAuthCFS_flg] -> DTC_Info/3
  DTC_Info/1 -> VDDM_KeyAuthDTC_raw32/1  "VDDM_KeyAuthDTC_raw32"
  [VDDM_KeyAuthCFS_flg] -> SR_Latch3/2
  [VDDM_KeyAuthDet_flg] -> DTC_Info/1
  Constant38/1 -> Test Detection Criteria/4
  [DTC_clear_request] -> DTC_Info/4
  [DTC_clear_request] -> Switch6/2
  Switch6/1 -> Test Detection Criteria/1
  Switch5/1 -> [VDDM_xxx_flg], Switch6/3
  Constant2/1 -> Switch6/1
  [VDDM_xxx_flg] -> SR_Latch1/2(reset)

== system ddm/DDM/DDM/PMM/LV ==
  task_time_s : Inport
  VPMM_PwrStaSW_enum : Inport  Port=2
  VPMM_PowerSta_enum : Inport  Port=3
  VINP_LVBattDet12V_V : Inport  Port=4
  VINP_CANMsgValidBMS2_flg : Inport  Port=5
  DTC_clear_request : Inport  Port=6
  Initial LV battery voltage too low : Subsystem
  LV power supply voltage too high : Subsystem
  LV power supply voltage too low : Subsystem
  VDDM_IniLVLoDTC_raw32 : Outport
  VDDM_LVSupLoDTC_raw32 : Outport  Port=2
  VDDM_LVSupHiDTC_raw32 : Outport  Port=3
  wires:
  VPMM_PowerSta_enum/1 -> [VPMM_PowerSta_enum]
  VPMM_PwrStaSW_enum/1 -> [VPMM_PwrStaSW_enum]
  task_time_s/1 -> [task_time_s]
  VINP_LVBattDet12V_V/1 -> [VINP_LVBattDet12V_V]
  VINP_CANMsgValidBMS2_flg/1 -> [VINP_CANMsgValidBMS2_flg]
  [task_time_s] -> Initial LV battery voltage too low/1(task_time_s)
  [VINP_LVBattDet12V_V] -> Initial LV battery voltage too low/4(VINP_LVBattDet12V_V)
  [VINP_CANMsgValidBMS2_flg] -> Initial LV battery voltage too low/5(VINP_CANMsgValidBMS2_flg)
  [DTC_clear_request] -> Initial LV battery voltage too low/6(DTC_clear_request)
  [VPMM_PwrStaSW_enum] -> Initial LV battery voltage too low/3(VPMM_PwrStaSW_enum)
  [VPMM_PowerSta_enum] -> Initial LV battery voltage too low/2(VPMM_PowerSta_enum)
  Initial LV battery voltage too low/1(VDDM_IniLVLoDTC_raw32) -> VDDM_IniLVLoDTC_raw32/1
  [VPMM_PowerSta_enum] -> LV power supply voltage too low/2(VPMM_PowerSta_enum)
  [VPMM_PwrStaSW_enum] -> LV power supply voltage too low/3(VPMM_PwrStaSW_enum)
  [DTC_clear_request] -> LV power supply voltage too low/6(DTC_clear_request)
  [task_time_s] -> LV power supply voltage too low/1(task_time_s)
  LV power supply voltage too low/1(VDDM_LVSupLoDTC_raw32) -> VDDM_LVSupLoDTC_raw32/1
  [VINP_CANMsgValidBMS2_flg] -> LV power supply voltage too low/5(VINP_CANMsgValidBMS2_flg)
  [VINP_LVBattDet12V_V] -> LV power supply voltage too low/4(VINP_LVBattDet12V_V)
  [task_time_s] -> LV power supply voltage too high/1(task_time_s)
  [VPMM_PwrStaSW_enum] -> LV power supply voltage too high/3(VPMM_PwrStaSW_enum)
  [VINP_CANMsgValidBMS2_flg] -> LV power supply voltage too high/5(VINP_CANMsgValidBMS2_flg)
  [VPMM_PowerSta_enum] -> LV power supply voltage too high/2(VPMM_PowerSta_enum)
  [VINP_LVBattDet12V_V] -> LV power supply voltage too high/4(VINP_LVBattDet12V_V)
  [DTC_clear_request] -> LV power supply voltage too high/6(DTC_clear_request)
  LV power supply voltage too high/1(VDDM_LVSupHiDTC_raw32) -> VDDM_LVSupHiDTC_raw32/1
  DTC_clear_request/1 -> [DTC_clear_request]

== system ddm/DDM/DDM/PMM/SW failure ==
  task_time_s : Inport
  VPMM_PwrStaSW_enum : Inport  Port=2
  VPMM_PowerSta_enum : Inport  Port=3
  DTC_clear_request : Inport  Port=4
  VINP_DrStSW : Inport  Port=5
  VINP_FLAJARSW : Inport  Port=6
  VINP_FRAJARSW : Inport  Port=7
  VINP_RLAJARSW : Inport  Port=8
  VINP_RRAJARSW : Inport  Port=9
  VINP_HoodSW : Inport  Port=10
  VINP_TailgaSW : Inport  Port=11
  Driver seat switch failure : Subsystem
  FL Door switch failure : Subsystem
  FR Door switch failure : Subsystem
  Hood switch failure : Subsystem
  RL Door switch failure : Subsystem
  RR Door switch failure : Subsystem
  Tailgate switch failure : Subsystem
  VDDM_DrStSWDTC_raw32 : Outport
  VDDM_FLDoorSWDTC_raw32 : Outport  Port=2
  VDDM_RLDoorSWDTC_raw32 : Outport  Port=3
  VDDM_FRDoorSWDTC_raw32 : Outport  Port=4
  VDDM_RRDoorSWDTC_raw32 : Outport  Port=5
  VDDM_HoodSWDTC_raw32 : Outport  Port=6
  VDDM_TailgaSWDTC_raw32 : Outport  Port=7
  Dr_SeatSta : Outport  Port=8
  VCUFLDoorSta : Outport  Port=9
  VCUFRDoorSta : Outport  Port=10
  VCURLDoorSta : Outport  Port=11
  VCURRDoorSta : Outport  Port=12
  VCUHoodSWSta : Outport  Port=13
  VCUTailgaSWSta : Outport  Port=14
  wires:
  Driver seat switch failure/1(VDDM_DrStSWDTC_raw32) -> VDDM_DrStSWDTC_raw32/1
  [VPMM_PowerSta_enum] -> Driver seat switch failure/2(VPMM_PowerSta_enum)
  [VPMM_PwrStaSW_enum] -> Driver seat switch failure/3(VPMM_PwrStaSW_enum)
  [DTC_clear_request] -> Driver seat switch failure/5(DTC_clear_request)
  [VINP_DrStSW] -> Driver seat switch failure/4(VINP_DrStSW)
  [task_time_s] -> Driver seat switch failure/1(task_time_s)
  VINP_DrStSW/1 -> [VINP_DrStSW]
  task_time_s/1 -> [task_time_s]
  VPMM_PwrStaSW_enum/1 -> [VPMM_PwrStaSW_enum]
  VPMM_PowerSta_enum/1 -> [VPMM_PowerSta_enum]
  DTC_clear_request/1 -> [DTC_clear_request]
  Driver seat switch failure/2(Dr_SeatSta) -> Dr_SeatSta/1
  VINP_FLAJARSW/1 -> [VINP_FLAJARSW]
  VINP_FRAJARSW/1 -> [VINP_FRAJARSW]
  VINP_RLAJARSW/1 -> [VINP_RLAJARSW]
  VINP_RRAJARSW/1 -> [VINP_RRAJARSW]
  [task_time_s] -> FL Door switch failure/1(task_time_s)
  [VPMM_PowerSta_enum] -> FL Door switch failure/2(VPMM_PowerSta_enum)
  [VPMM_PwrStaSW_enum] -> FL Door switch failure/3(VPMM_PwrStaSW_enum)
  [VINP_FLAJARSW] -> FL Door switch failure/4(VINP_FLAJARSW)
  [DTC_clear_request] -> FL Door switch failure/5(DTC_clear_request)
  FL Door switch failure/1(VDDM_FLDoorSWDTC_raw32) -> VDDM_FLDoorSWDTC_raw32/1
  FL Door switch failure/2(VCUFLDoorSta) -> VCUFLDoorSta/1
  [task_time_s] -> FR Door switch failure/1(task_time_s)
  [VPMM_PowerSta_enum] -> FR Door switch failure/2(VPMM_PowerSta_enum)
  [VPMM_PwrStaSW_enum] -> FR Door switch failure/3(VPMM_PwrStaSW_enum)
  [VINP_FRAJARSW] -> FR Door switch failure/4(VINP_FRAJARSW)
  [DTC_clear_request] -> FR Door switch failure/5(DTC_clear_request)
  FR Door switch failure/1(VDDM_FRDoorSWDTC_raw32) -> VDDM_FRDoorSWDTC_raw32/1
  FR Door switch failure/2(VCUFRDoorSta) -> VCUFRDoorSta/1
  [VPMM_PwrStaSW_enum] -> RL Door switch failure/3(VPMM_PwrStaSW_enum)
  [VPMM_PowerSta_enum] -> RL Door switch failure/2(VPMM_PowerSta_enum)
  [task_time_s] -> RL Door switch failure/1(task_time_s)
  [VINP_RLAJARSW] -> RL Door switch failure/4(VINP_RLAJARSW)
  [DTC_clear_request] -> RL Door switch failure/5(DTC_clear_request)
  RL Door switch failure/1(VDDM_RLDoorSWDTC_raw32) -> VDDM_RLDoorSWDTC_raw32/1
  RL Door switch failure/2(VCURLDoorSta) -> VCURLDoorSta/1
  [task_time_s] -> RR Door switch failure/1(task_time_s)
  [VPMM_PowerSta_enum] -> RR Door switch failure/2(VPMM_PowerSta_enum)
  [VPMM_PwrStaSW_enum] -> RR Door switch failure/3(VPMM_PwrStaSW_enum)
  [VINP_RRAJARSW] -> RR Door switch failure/4(VINP_RRAJARSW)
  [DTC_clear_request] -> RR Door switch failure/5(DTC_clear_request)
  RR Door switch failure/1(VDDM_RRDoorSWDTC_raw32) -> VDDM_RRDoorSWDTC_raw32/1
  RR Door switch failure/2(VCURRDoorSta) -> VCURRDoorSta/1
  [task_time_s] -> Hood switch failure/1(task_time_s)
  [VPMM_PowerSta_enum] -> Hood switch failure/2(VPMM_PowerSta_enum)
  [VPMM_PwrStaSW_enum] -> Hood switch failure/3(VPMM_PwrStaSW_enum)
  VINP_HoodSW/1 -> [VINP_HoodSW]
  VINP_TailgaSW/1 -> [VINP_TailgaSW]
  [VINP_HoodSW] -> Hood switch failure/4(VINP_HoodSW)
  [DTC_clear_request] -> Hood switch failure/5(DTC_clear_request)
  Hood switch failure/1(VDDM_HoodSWDTC_raw32) -> VDDM_HoodSWDTC_raw32/1
  Hood switch failure/2(VCUHoodSWSta) -> VCUHoodSWSta/1
  [task_time_s] -> Tailgate switch failure/1(task_time_s)
  [VPMM_PowerSta_enum] -> Tailgate switch failure/2(VPMM_PowerSta_enum)
  [VPMM_PwrStaSW_enum] -> Tailgate switch failure/3(VPMM_PwrStaSW_enum)
  [DTC_clear_request] -> Tailgate switch failure/5(DTC_clear_request)
  [VINP_TailgaSW] -> Tailgate switch failure/4(VINP_TailgaSW)
  Tailgate switch failure/1(VDDM_TailgaSWDTC_raw32) -> VDDM_TailgaSWDTC_raw32/1
  Tailgate switch failure/2(VCUTailgaSWSta) -> VCUTailgaSWSta/1

== system ddm/DDM/DDM/PMM/System conditions of ON to READY not satisfied ==
  note: Release Condition During Failure Detection
  note: Fail Safe Operation After Failure Decision
  note: Test Detection Criteria
  note: Release Condition After Failure Decision
  note: Diagnostics and Fault Handling
  note: Test Pass Criteria
  note: Fail Safe Operation During Failure Detection
  task_time_s : Inport
  VPMM_PowerSta_enum : Inport  Port=2
  VPMM_PwrStaSW_enum : Inport  Port=3
  VDDM_BrakeSW_enum : Inport  Port=4
  DTC_clear_request : Inport  Port=5
  VPMM_MCUReady_flg : Inport  Port=6
  VINP_AllowMovThd_OTA_enum : Inport  Port=7
  VDHP_EAPS12RangeSta_enum : Inport  Port=8
  VDDM_KeyAuthDTC_raw32 : Inport  Port=9
  Constant : Constant  Value=ENUM_RANGESTA_12OUT
  Constant1 : Constant  Value=ENUM_ALLOWMOV_ALLOWREADY
  Constant11 : Constant  Value=KDDM_ONtoRdyPassSW_flg
  Constant15 : Constant  Value=KDDM_ONtoRdyCFSSW_flg
  Constant16 : Constant  Value=TRUE
  Constant19 : Constant  Value=ENUM_POWERSTA_OFF
  Constant{2,21,25,27} (4 alike) : Constant  Value=FALSE
  Constant20 : Constant  Value=KDDM_ONtoRdyDFSSW_flg
  Constant23 : Constant  Value=TRUE
  Constant24 : Constant  Value=TRUE
  Constant26 : Constant  Value=ENUM_PWRSTASW_READY
  Constant3 : Constant  Value=ENUM_BRKSTA_ON
  Constant38 : Constant  Value=KDDM_ONtoRdyDetTO_s
  Constant4 : Constant  Value=ENUM_PWRSTASW_READY
  Constant40 : Constant  Value=KDDM_ONtoRdyDTC_cnt
  Constant43 : Constant  Value=KDDM_ONtoRdyPassTO_s
  Constant44 : Constant  Value=KDDM_ONtoRdyDetSW_flg
  Constant5 : Constant  Value=ENUM_BRKSTA_ON
  Constant6 : Constant  Value=ENUM_ALLOWMOV_ALLOWREADY
  Constant7 : Constant  Value=KDDM_ONtoRdyPassTO_s
  Constant8 : Constant  Value=KDDM_ONtoRdyDTC_cnt
  Constant9 : Constant  Value=ENUM_RANGESTA_12OUT
  DTC_Couter : hcu_lib/Basic_Blocks/DTC_Couter
  DTC_Info : hcu_lib/Basic_Blocks/DTC_Info
  Data Type Conversion1 : DataTypeConversion  OutDataTypeStr=uint8
  Data Type Conversion28 : DataTypeConversion  OutDataTypeStr=boolean
  Equal{,2..3,5..7,9} (7 alike) : RelationalOperator  Operator===  OutDataTypeStr=boolean  RndMeth=Simplest
  Equal1 : RelationalOperator  Operator=~=  OutDataTypeStr=boolean  RndMeth=Simplest
  Equal4 : RelationalOperator  OutDataTypeStr=boolean  RndMeth=Simplest
  Equal8 : RelationalOperator  Operator=~=  OutDataTypeStr=boolean  RndMeth=Simplest
  Logical Operator : Logic  Operator=NOT  AllPortsSameDT=off  OutDataTypeStr=boolean
  Logical Operator{1..2,12,15,18..19} (6 alike) : Logic  AllPortsSameDT=off  OutDataTypeStr=boolean
  Logical Operator3 : Logic  Operator=OR  AllPortsSameDT=off  OutDataTypeStr=boolean
  Logical Operator4 : Logic  Operator=OR  Inputs=4  AllPortsSameDT=off  OutDataTypeStr=boolean
  Logical Operator5 : Logic  Operator=NOT  AllPortsSameDT=off  OutDataTypeStr=boolean
  Logical Operator6 : Logic  Operator=NOT  AllPortsSameDT=off  OutDataTypeStr=boolean
  Logical Operator7 : Logic  Operator=OR  Inputs=4  AllPortsSameDT=off  OutDataTypeStr=boolean
  Logical Operator8 : Logic  Operator=OR  AllPortsSameDT=off  OutDataTypeStr=boolean
  Relay : Relay  OnSwitchValue=ONE_INT  OffSwitchValue=ZERO_INT
  SR_Latch1 : Subsystem  mask(SR_Latch){}
      mask help: SR latch function.
  SR_Latch3 : hcu_lib/Basic_Blocks/SR_Latch
  SR_Latch4 : hcu_lib/Basic_Blocks/SR_Latch
  Switch{,2,4..6} (5 alike) : Switch  Criteria=u2 ~= 0
  Test Detection Criteria : hcu_lib/Basic_Blocks/Test Detection Criteria
  Timer1 : hcu_lib/Basic_Blocks/Timer
  VDDM_ONtoRdyDTC_raw32 : Outport
  VDDM_EDriveSysErrONtoRdy_flg : Outport  Port=2
  VDDM_SysAllowReadySta_flg : Outport  Port=3
  wires:
  DTC_clear_request/1 -> [DTC_clear_request]
  Constant4/1 -> Equal3/2
  Equal6/1 -> Logical Operator1/2
  Constant5/1 -> Equal6/2
  [VDDM_BrakeSW_enum] -> Equal6/1
  Logical Operator1/1 -> Switch2/2
  Equal3/1 -> Logical Operator1/1
  [VPMM_PwrStaSW_enum] -> Equal3/1
  Constant3/1 -> Equal2/2
  [VDDM_BrakeSW_enum] -> Equal2/1
  Equal2/1 -> Logical Operator2/2
  [DTC_clear_request] -> Logical Operator8/2
  [VDDM_ONtoRdyCFSRls_flg] -> SR_Latch4/2
  Equal5/1 -> Logical Operator8/1
  SR_Latch3/1 -> Logical Operator12/2
  Constant23/1 -> Switch2/3
  Constant7/1 -> Equal4/2
  Constant44/1 -> Logical Operator19/2
  Equal4/1 -> SR_Latch1/1(set)
  Constant25/1 -> Switch4/3
  Constant8/1 -> DTC_Couter/3
  SR_Latch4/1 -> Logical Operator18/1
  Test Detection Criteria/1 -> [VDDM_ONtoRdyDet_flg]  "VDDM_ONtoRdyDet_flg"
  Constant20/1 -> Logical Operator12/1
  Constant21/1 -> Switch/3
  Relay/1 -> SR_Latch3/1
  [VDDM_ONtoRdyDet_flg] -> Logical Operator19/1
  Switch4/1 -> [VDDM_ONtoRdyCFSRls_flg]
  Logical Operator8/1 -> Switch4/2
  Constant19/1 -> Equal5/2
  DTC_Couter/1 -> SR_Latch4/1
  Logical Operator2/1 -> Switch5/2
  Constant16/1 -> Switch/1
  [VPMM_PowerSta_enum] -> Equal5/1
  [VDDM_ONtoRdyPass_flg] -> Logical Operator3/1
  DTC_Couter/2 -> Data Type Conversion1/1
  Switch/1 -> [VDDM_SysAllowReadySta_flg], [VDDM_EDriveSysErrONtoRdy_flg]  "VDDM_SysAllowReadySta_flg"
  [VDDM_ONtoRdyCFSRls_flg] -> Logical Operator3/2
  Logical Operator18/1 -> [VDDM_ONtoRdyCFS_flg]
  Switch2/1 -> Logical Operator6/1, Timer1/2
  Equal/1 -> Logical Operator2/1
  Logical Operator19/1 -> DTC_Couter/1
  Constant24/1 -> Switch4/1
  Constant27/1 -> Switch5/3
  [VDDM_ONtoRdyCFS_flg] -> Switch/2
  SR_Latch1/1(latched) -> [VDDM_ONtoRdyPass_flg]
  Logical Operator12/1 -> [VDDM_ONtoRdyDFS_flg]
  Logical Operator6/1 -> Timer1/1
  Logical Operator15/1 -> DTC_Couter/2
  Data Type Conversion1/1 -> [VDDM_ONtoRdyDTC_cnt]  "VDDM_ONtoRdyDTC_cnt"
  Constant11/1 -> Logical Operator15/2
  Constant15/1 -> Logical Operator18/2
  Constant26/1 -> Equal/2
  Constant43/1 -> Timer1/4
  Constant40/1 -> Test Detection Criteria/3
  Logical Operator3/1 -> Logical Operator15/1
  [VDDM_ONtoRdyDTC_cnt] -> Relay/1
  [task_time_s] -> Test Detection Criteria/2
  [VPMM_PwrStaSW_enum] -> Equal/1
  Timer1/1 -> Equal4/1
  VDDM_BrakeSW_enum/1 -> [VDDM_BrakeSW_enum]
  task_time_s/1 -> [task_time_s]
  VPMM_PwrStaSW_enum/1 -> [VPMM_PwrStaSW_enum]
  VPMM_PowerSta_enum/1 -> [VPMM_PowerSta_enum]
  VPMM_MCUReady_flg/1 -> [VPMM_MCUReady_flg]
  VINP_AllowMovThd_OTA_enum/1 -> [VINP_AllowMovThd_OTA_enum]
  VDHP_EAPS12RangeSta_enum/1 -> [VDHP_EAPS12RangeSta_enum]
  [VPMM_MCUReady_flg] -> Logical Operator/1
  [VINP_AllowMovThd_OTA_enum] -> Equal1/1
  Constant1/1 -> Equal1/2
  [VDHP_EAPS12RangeSta_enum] -> Equal7/1
  Constant/1 -> Equal7/2
  Logical Operator/1 -> Logical Operator4/1
  Equal1/1 -> Logical Operator4/2
  Equal7/1 -> Logical Operator4/3
  [VDDM_KeyAuthCFS_flg] -> Logical Operator4/4
  Logical Operator4/1 -> Switch5/1
  [VDDM_KeyAuthCFS_flg] -> Logical Operator7/4
  Equal9/1 -> Logical Operator7/3
  Equal8/1 -> Logical Operator7/2
  Logical Operator5/1 -> Logical Operator7/1
  Constant9/1 -> Equal9/2
  [VDHP_EAPS12RangeSta_enum] -> Equal9/1
  Constant6/1 -> Equal8/2
  [VINP_AllowMovThd_OTA_enum] -> Equal8/1
  [VPMM_MCUReady_flg] -> Logical Operator5/1
  Logical Operator7/1 -> Switch2/1
  [VDDM_EDriveSysErrONtoRdy_flg] -> VDDM_EDriveSysErrONtoRdy_flg/1
  [VDDM_SysAllowReadySta_flg] -> VDDM_SysAllowReadySta_flg/1
  [task_time_s] -> Timer1/3
  DTC_Info/1 -> VDDM_ONtoRdyDTC_raw32/1  "VDDM_ONtoRdyDTC_raw32"
  [VDDM_ONtoRdyPass_flg] -> DTC_Info/2
  [VDDM_ONtoRdyCFS_flg] -> DTC_Info/3
  [VDDM_ONtoRdyCFS_flg] -> SR_Latch3/2
  VDDM_KeyAuthDTC_raw32/1 -> Data Type Conversion28/1
  Data Type Conversion28/1 -> [VDDM_KeyAuthCFS_flg]
  [VDDM_ONtoRdyDet_flg] -> DTC_Info/1
  Constant38/1 -> Test Detection Criteria/4
  [DTC_clear_request] -> DTC_Info/4
  [DTC_clear_request] -> Switch6/2
  Switch6/1 -> Test Detection Criteria/1
  Switch5/1 -> [VDDM_xxxx_flg], Switch6/3
  Constant2/1 -> Switch6/1
  [VDDM_xxxx_flg] -> SR_Latch1/2(reset)
